simulink model "buoy_lowpowerdc"  (R2025a)
settings: Solver=VariableStepAuto  StartTime=0.0  StopTime=100  RelTol=1e-3
undefined symbols (not defined in the file): magnitude, ptoSim, simu
libraries: fl_lib x6, nesl_utility x4, ee_lib x1
settings Model: Creator=jacks  LastModifiedBy=jacks

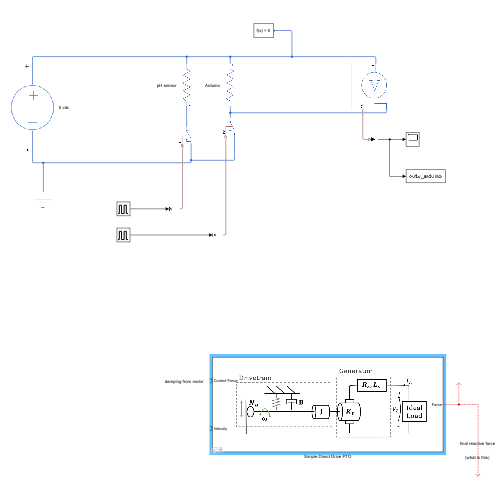
[thumbnail: Simulink's stored preview of the top-level diagram]
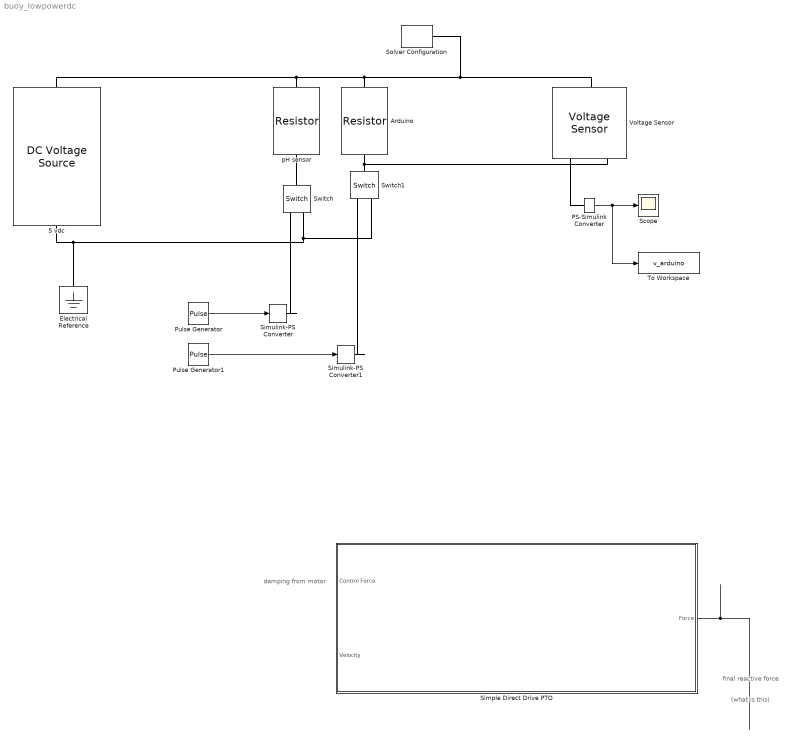
== system buoy_lowpowerdc ==
  note: (what is this)
  note: damping from motor
  note: final reactive force
  5 vdc : ee_lib/Additional Components/SPICE Sources/DC Voltage Source  DC=5 V
  Arduino : fl_lib/Electrical/Electrical Elements/Resistor  R=4 Ohm  i_specify=off  i_priority=None  i=0 A  i_nominal_specify=off  i_nominal_value=1  i_nominal_unit=A  v_specify=off  v_priority=None  v=0 V  v_nominal_specify=off  v_nominal_value=1  v_nominal_unit=V
  Electrical Reference : fl_lib/Electrical/Electrical Elements/Electrical Reference
  PS-Simulink Converter : nesl_utility/PS-Simulink Converter  PhysicalDomain=network_engine_domain  SubClassName=ps_output  LeftPortType=input  RightPortType=output  PseudoPeriodic=off  Frequencies=[]  VectorFormat=inherit  Unit=inherit  AffineConversion=off
  Pulse Generator : DiscretePulseGenerator  PulseType=Time based  Period=10  PulseWidth=50
  Pulse Generator1 : DiscretePulseGenerator  PulseType=Time based  Period=10  PulseWidth=70
  Scope : Scope
      settings: ActiveDisplayYMinimum=-3.6194258251400333  ActiveDisplayYMaximum=9.34147252926366
  Simple Direct Drive PTO : Subsystem  AncestorBlock=WECSim_Lib_PTOSim/Electric/Simple Direct Drive PTO  mask{ptoSim=ptoSim(1)}
      mask prompts: ptoSim "Simple Direct Drive PTO"
      mask init:
      | if exist('ptoSim', 'var')
      |     h=[gcb '/To Workspace'];
      |     responseName=['ptoSim' num2str(ptoSim.number) '_out'];
      |     set_param(h,'VariableName',responseName);
      | end
      | clear h responseName
      mask Display: image('simpleDDPTO.png'); % Use "Edit Image" on toolstrip to change.
  Simulink-PS Converter : nesl_utility/Simulink-PS Converter  PhysicalDomain=network_engine_domain  SubClassName=ps_input  LeftPortType=input  RightPortType=output  PseudoPeriodic=off  Frequencies=[]  NoiseDistribution=none  NoiseParameters=[]  Unit=1  AffineConversion=off  FilteringAndDerivatives=provide  SimscapeFilterOrder=1  InputFilterTimeConstant=0.001  UdotUserProvided=0
  Simulink-PS Converter1 : nesl_utility/Simulink-PS Converter  PhysicalDomain=network_engine_domain  SubClassName=ps_input  LeftPortType=input  RightPortType=output  PseudoPeriodic=off  Frequencies=[]  NoiseDistribution=none  NoiseParameters=[]  Unit=1  AffineConversion=off  FilteringAndDerivatives=provide  SimscapeFilterOrder=1  InputFilterTimeConstant=0.001  UdotUserProvided=0
  Solver Configuration : nesl_utility/Solver Configuration  PhysicalDomain=network_engine_domain  SubClassName=solver  LeftPortType=input  RightPortType=generic  Tones=[]  Harmonics=[]  SimulateNoise=off  Profile=off  UseLocalSampling=off  EnableSwitchedLinearOptims=on  FrequencyDomain=off  UseCCode=off  RelTol=0.001  AbsTol=0.001  MinStep=1e-09  ToWorkspace=off  RevertToSquareIcSolve=off  NumHomotopyIterations=100  PhasorMode=off  PhasorModeNumHarmonics=1  ConsistencySolver=NEWTON_XTOL_AFTER_FTOL  IndexReductionMethod=DerivativeReplacement  DoDC=off  ResidualTolerance=1e-09  ConsistencyTolSource=GLOBAL  ConsistencyAbsTol=0.001  ConsistencyRelTol=0.001  ConsistencyTolFactor=0.001  UseLocalSolver=off  LocalSolverChoice=NE_BACKWARD_EULER_ADVANCER  ResolveIndetEquations=on  FunctionEvalNumThread=1  LocalSolverSampleTime=0.001  DoFixedCost=off  MaxNonlinIter=3  MaxModeIter=2  ComputeImpulses=off  ImpulseIterations=2  LinearAlgebra=auto  LinearAlgebraNumThread=0  EquationFormulation=NE_TIME_EF  DelaysMemoryBudget=1024  AutomaticFiltering=on  FilteringTimeConstant=0.001  PartitionStorageMethod=AS_NEEDED  PartitionMemoryBudget=1024  PartitionMethod=ROBUST  MultibodyUseLocalSolver=off  MultibodyLocalSolverChoice=ODE1  MultibodyLocalSolverSampleTime=0.001
  Switch : fl_lib/Electrical/Electrical Elements/Switch  R_closed=0.01 Ohm  G_open=1e-8 1/Ohm  Threshold=0.5  i_specify=off  i_priority=None  i=0 A  i_nominal_specify=off  i_nominal_value=1  i_nominal_unit=A  v_specify=off  v_priority=None  v=0 V  v_nominal_specify=off  v_nominal_value=1  v_nominal_unit=V
  Switch1 : fl_lib/Electrical/Electrical Elements/Switch  R_closed=0.01 Ohm  G_open=1e-8 1/Ohm  Threshold=0.5  i_specify=off  i_priority=None  i=0 A  i_nominal_specify=off  i_nominal_value=1  i_nominal_unit=A  v_specify=off  v_priority=None  v=0 V  v_nominal_specify=off  v_nominal_value=1  v_nominal_unit=V
  To Workspace : ToWorkspace  VariableName=v_arduino  SaveFormat=Timeseries  SampleTime=-1
  Voltage Sensor : fl_lib/Electrical/Electrical Sensors/Voltage Sensor
  pH sensor : fl_lib/Electrical/Electrical Elements/Resistor  R=1 Ohm  i_specify=off  i_priority=None  i=0 A  i_nominal_specify=off  i_nominal_value=1  i_nominal_unit=A  v_specify=off  v_priority=None  v=0 V  v_nominal_specify=off  v_nominal_value=1  v_nominal_unit=V
  wires:
  Pulse Generator/1 -> Simulink-PS Converter/1
  Pulse Generator1/1 -> Simulink-PS Converter1/1
  PS-Simulink Converter/1 -> To Workspace/1, Scope/1
  Simple Direct Drive PTO/1(Force) -> ?
  connections:
  5 vdc/LConn1 -- Solver Configuration/RConn1 -- Voltage Sensor/LConn1 -- Arduino/LConn1 -- pH sensor/LConn1
  5 vdc/RConn1 -- Electrical Reference/LConn1 -- Switch1/RConn2 -- Switch/RConn2
  Switch/LConn1 -- pH sensor/RConn1
  Simulink-PS Converter/RConn1 -- Switch/RConn1
  Switch1/LConn1 -- Voltage Sensor/RConn2 -- Arduino/RConn1
  Simulink-PS Converter1/RConn1 -- Switch1/RConn1
  Voltage Sensor/RConn1 -- PS-Simulink Converter/LConn1

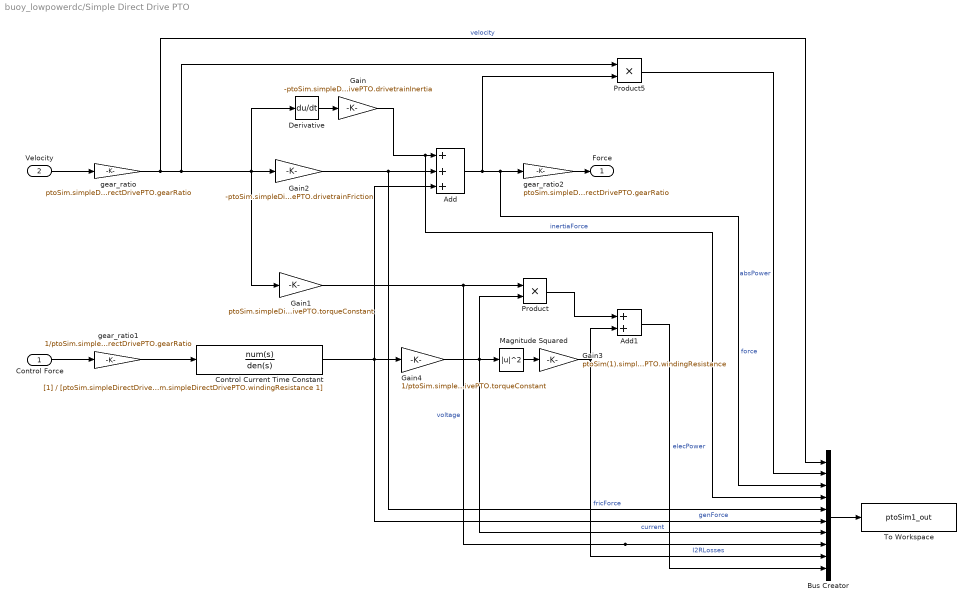
== system buoy_lowpowerdc/Simple Direct Drive PTO ==
  Control Force : Inport
  Velocity : Inport  Port=2
  Add : Sum  Inputs=+++
  Add1 : Sum
  Bus Creator : BusCreator  Inputs=10
  Control Current Time Constant : TransferFcn  Denominator=[ptoSim.simpleDirectDrivePTO.windingInductance/ptoSim.simpleDirectDrivePTO.windingResistance 1]
  Derivative : Derivative  CoefficientInTFapproximation=1000*2*pi
  Gain : Gain  Gain=-ptoSim.simpleDirectDrivePTO.drivetrainInertia
  Gain1 : Gain  Gain=ptoSim.simpleDirectDrivePTO.torqueConstant
  Gain2 : Gain  Gain=-ptoSim.simpleDirectDrivePTO.drivetrainFriction
  Gain3 : Gain  Gain=ptoSim(1).simpleDirectDrivePTO.windingResistance
  Gain4 : Gain  Gain=1/ptoSim.simpleDirectDrivePTO.torqueConstant
  Magnitude Squared : Math  Operator=magnitude^2
  Product : Product
  Product5 : Product
  To Workspace : ToWorkspace  VariableName=ptoSim1_out  SaveFormat=Structure With Time  SampleTime=simu.dtOut
  gear_ratio : Gain  Gain=ptoSim.simpleDirectDrivePTO.gearRatio
  gear_ratio1 : Gain  Gain=1/ptoSim.simpleDirectDrivePTO.gearRatio
  gear_ratio2 : Gain  Gain=ptoSim.simpleDirectDrivePTO.gearRatio
  Force : Outport
  wires:
  gear_ratio2/1 -> Force/1
  gear_ratio1/1 -> Control Current Time Constant/1
  gear_ratio/1 -> Product5/1, Derivative/1, Gain2/1, Gain1/1, Bus Creator/1  "velocity"
  Add1/1 -> Bus Creator/10  "elecPower"
  Add/1 -> Product5/2, Bus Creator/3, gear_ratio2/1  "force"
  Gain3/1 -> Bus Creator/9, Add1/2  "I2RLosses"
  Product5/1 -> Bus Creator/2  "absPower"
  Gain4/1 -> Bus Creator/7, Product/2, Magnitude Squared/1  "current"
  Bus Creator/1 -> To Workspace/1
  Gain2/1 -> Bus Creator/5, Add/2  "fricForce"
  Gain1/1 -> Bus Creator/8, Product/1  "voltage"
  Product/1 -> Add1/1
  Magnitude Squared/1 -> Gain3/1
  Velocity/1 -> gear_ratio/1
  Control Current Time Constant/1 -> Bus Creator/6, Add/3, Gain4/1  "genForce"
  Gain/1 -> Add/1, Bus Creator/4  "inertiaForce"
  Control Force/1 -> gear_ratio1/1
  Derivative/1 -> Gain/1
